simulink library "HANcoder_STM32_Target"  (R2018b)
settings: Solver=ode45  StartTime=0.0  StopTime=10.0  RelTol=1e-3  EnableMultiTasking=on
libraries: simulink x4
(part 3 of 9)

== system HANcoder_STM32_Target/Olimexino STM32 F3/PWM Outputs ==
  PWM Duty Cycle : Subsystem  Tag=HANcoder_TARGET_STM32_F3_Olimexino  mask(Pulse Width Modulation Set Duty Cycle){pinID=TIM1 - CON3 - D6, tsamp=-1}
      mask prompts: pinID "Output pin"; tsamp "Sample time"
      mask help:
      | Function
      | ========
      | A 'PWM Duty Cycle' block allows the duty cycle of the generated PWM signal to
      | changed.
      | Note that this only works properly if a 'PWM Init' block is also present
      | for initializing the related PWM module.
      |
      | Parameters
      | ==========
      | PWM pin:
      |   Selects the PWM pin for which the duty cycle should be updated.
      |
      | Inport
      | ==========
      | uint16 10-bit unsigned value (0..1023) to represent the duty cycle (0..100%) for
      | each enabled channel.
      mask init:
      | pinIDInfoStr = sfcn_pwmout_setduty_mcb(1, pinID);
      settings: MoveFcn=drawLogos
      mask Help: web('sfcn_pwmout_setduty.html');
      mask TypeOptions pinID: TIM1 - CON3 - D6 | TIM1 - CON3 - D7 | TIM1 - CON4 - D8 | TIM2 - CON3 - D2 | TIM2 - CON3 - D3 | TIM2 - CON3 - D0 | TIM3 - EXT - D35 | TIM3 - EXT - D36 | TIM3 - EXT - D37 | TIM4 - CON3 - D5 | TIM4 - CON4 - D9 | TIM4 - CON4 - D14 | TIM4 - EXT - D24
      mask Display: fprintf('PWM Set Duty Cycle\n%s', pinIDInfoStr);patch([129 148 147 128],[2 6 10 6],[0.89804 0 0.33725]);
  PWM Frequency : Subsystem  Tag=HANcoder_TARGET_STM32_F3_Olimexino  mask(Pulse Width Modulation Set Frequency){timID=TIM1, tsamp=-1}
      mask prompts: timID "Select a timer"; tsamp "Sample time"
      mask help:
      | Function
      | ========
      | A 'PWM Frequency' block allows the frequency of the generated PWM signal to change.
      | Note that this only works properly if a 'PWM Init' block is also present for initializing the related PWM module.
      |
      | Parameters
      | ==========
      | TIM:
      |   Selects the timer for which the frequency should be updated.
      |
      | Inport
      | ==========
      | A value that represents the new frequency [Hz]
      mask init:
      | timIDInfoStr = sfcn_pwmout_setfrequency_mcb(1, timID);
      settings: MoveFcn=drawLogos
      mask Help: web('sfcn_pwmout_setfrequency.html');
      mask TypeOptions timID: TIM1 | TIM2 | TIM3 | TIM4
      mask Display: fprintf('PWM Set frequency\n%s', timIDInfoStr);patch([129 148 147 128],[2 6 10 6],[0.89804 0 0.33725]);
  PWM Init : Subsystem  Tag=HANcoder_TARGET_STM32_F3_Olimexino  mask(Pulse Width Modulation Initialization){moduleID=TIM1: D6 & D7 & D8 & n/a + N-channels D32 & D33 & D34, frequency=5022, alignment=Edge aligned, enableIRQoutput=off, ch1On=off, ch1Pol=Active high, ch1Inv=off, ch2On=off, ch2Pol=Active high, ch2Inv=off, ch3On=off, ch3Pol=Active high, ch3Inv=off, ch4On=off, ch4Pol=Active high, ch4Inv=off}
      mask prompts: moduleID "PWM module"; frequency "Signal frequency [Hz]"; alignment "Signal alignment"; enableIRQoutput "Enable IRQ output"; ch1On "Generate PWM signal on channel 1"; ch1Pol "Select signal polarity"; ch1Inv "Enable inverted signal on additional output pin"; ch2On "Generate PWM signal on channel 2"; ch2Pol "Select signal polarity"; ch2Inv "Enable inverted signal on additional output pin"; ch3On "Generate PWM signal on channel 3"; ch3Pol "Select signal polarity"; ch3Inv "Enable inverted signal on additional output pin"; ch4On "Generate PWM signal on channel 4"; ch4Pol "Select signal polarity"; ch4Inv "Enable inverted signal on additional output pin"
      mask help:
      | Function
      | ========
      | A 'PWM Init' block configures one of the STM32 timer modules for PWM
      | functionality, allowing a PWM signal to be generated on up to 4 timer
      | channels and their associated output pins.
      |
      | Parameters
      | ==========
      | General - PWM module:
      |   Select the PWM module to use. The name in the combo box contains
      |   information about which pins on the target belong to this timer module.
      |   Also the first pin corresponds with the first channel and so on:
      |   TIMx: Ch1 & Ch2 & Ch3...
      |
      | General - Signal frequency:
      |   Determines the signal frequency in Hz. If you click 'Apply' after entering
      |   the desired frequency it will automatically be adjusted to the closest
      |   supported value.
      |
      | General - Signal Aligment:
      |   Determines the aligment of the signal. It can either be edge aligned or
      |   center aligned.
      |
      | General - Enable IRQ output
      |   Controls whether or not the IRQ output is available.
      |
      | Channel x - Generate PWM signal on channel x:
      |   Enable to configure the channel for PWM functionality so that the PWM signal
      |   is outputted on the channel's associated microcontroller pin.
      |
      | Channel x - Signal polarity:
      |   Selects the polarity of the signal.
      |
      | Channel x - Enable inverted signal on additional output pin:
      |   When enabled, a second PWM signal will be generated on an additional
      |   microcontroller pin where the signal is an exact inversion of the first signal.
      mask init:
      | moduleIDInfoStr = sfcn_pwmout_init_mcb(1, moduleID, frequency, alignment, enableIRQoutput, ch1On, ch2On, ch3On, ch4On, ch1Pol, ch2Pol, ch3Pol, ch4Pol, ch1Inv, ch2Inv, ch3Inv, ch4Inv);
      settings: CopyFcn=sfcn_pwmout_init_chk();  MoveFcn=drawLogos
      mask Help: web('sfcn_pwmout_init.html');
      mask TypeOptions moduleID: TIM1: D6 & D7 & D8 & n/a + N-channels D32 & D33 & D34  | TIM2: D2 & D3 & n/a & D0 | TIM3: D35 & D36 & D37 & n/a | TIM4: D5 & D9 & D14 & D24
      mask Callback moduleID: sfcn_pwmout_init_chk();
      mask TypeOptions alignment: Edge aligned | Center aligned
      mask TypeOptions ch1Pol: Active high | Active low
      mask TypeOptions ch2Pol: Active high | Active low
      mask TypeOptions ch3Pol: Active high | Active low
      mask TypeOptions ch4Pol: Active high | Active low
      mask Display: fprintf('PWM Init\n%s', moduleIDInfoStr);patch([214 233 232 213],[2 6 10 6],[0.89804 0 0.33725]);

== system HANcoder_STM32_Target/Olimexino STM32 F3/SPI ==
  SPI master init : Subsystem  Tag=HANcoder_TARGET_STM32_F3_Olimexino  mask(SPI master init){channel=SPI1: D13 & D12 & D11, speed=9000 kHz, polarity=Idle low, phase=Sample bit on 1st clock edge}
      mask prompts: speed "Communication speed"
      mask help:
      | Function
      | ==========
      | Initialized a SPI master channel.
      |
      | Parameters per channel
      | ======================
      | - Select channel (SCK MISO MOSI)
      | - Select communication speed
      | - Select clock signal polarity
      | - Select clock phase to sample a bit
      mask init:
      | spiChannelInfoStr = sfcn_spi_master_init_mcb(1, channel, speed, polarity, phase);
      settings: CopyFcn=sfcn_spi_master_init_chk();  MoveFcn=drawLogos
      mask Help: web('sfcn_spi_master_init.html')
      mask TypeOptions channel: SPI1: D13 & D12 & D11 | SPI2: D32 & D33 & D34
      mask Callback channel: sfcn_spi_master_init_chk();
      mask TypeOptions speed: 36000 kHz | 18000 kHz | 9000 kHz | 4500 kHz | 2250 kHz | 1125 kHz | 562.5 kHz | 281.25 kHz
      mask TypeOptions polarity: Idle low | Idle high
      mask TypeOptions phase: Sample bit on 1st clock edge | Sample bit on 2nd clock edge
      mask Display: fprintf('SPI master init\n%s', spiChannelInfoStr);patch([205 224 223 204],[2 6 10 6],[0.89804 0 0.33725]);
  SPI master transfer : Subsystem  Tag=HANcoder_TARGET_STM32_F3_Olimexino  Priority=1  mask(SPI master transfer){channel=SPI1: D13 & D12 & D11, useSS=off, SSpin=CON2 - A0, SSenable=on, SSdisable=on, delayCycles=0, userPriority=1, tsamp=-1}
      mask prompts: useSS "Use slave select output"; SSpin "Slave select output pin"; SSenable "Enable slave select before transfer"; SSdisable "Disable slave select after transfer"; delayCycles "Delay cycles between slave select enable and transfer"; userPriority "Priority (use to set order of byte transfer, lowest number is executed first)"; tsamp "Sample time"
      mask help:
      | Function
      | ==========
      | Performs a byte transfer via SPI.
      |
      | Parameters per channel
      | ======================
      | - Select channel
      | - Select if a Slave Select output should be controlled
      |   * Select the Slave Select digital output pin
      |   * Select if the Slave Select should be made logic low before the transfer
      |   * Select if the Slave Select should be made logic high after the transfer
      |   * Enter the number of CPU cycles to delay between Slave Select enable and the transfer
      |
      | Inputs
      | ======
      | The byte value to send to the slave.
      |
      | Outputs
      | =======
      | The byte value received from the slave.
      mask init:
      | spiChannelInfoStr = sfcn_spi_master_transfer_mcb(1, channel, useSS, SSpin, SSenable, SSdisable, delayCycles);
      settings: MoveFcn=drawLogos
      mask Help: web('sfcn_spi_master_transfer.html')
      mask TypeOptions channel: SPI1: D13 & D12 & D11 | SPI2: D32 & D33 & D34
      mask Callback useSS:
      | % Get the mask parameter
      | useSS = get_param(gcb,'useSS');
      | 
      | if strcmp(useSS,'on')
      |     set_param(gcb,'MaskVisibilities',{'on','on','on','on','on','on','on','on'});
      | else
      |     set_param(gcb,'MaskVisibilities',{'on','on','off','off','off','off','on','on'});
      | end
      mask TypeOptions SSpin: CON2 - A0 | CON2 - A1 | CON2 - A2 | CON2 - A3 | CON2 - A4 | CON2 - A5 | CON3 - D0 | CON3 - D1 | CON3 - D2 | CON3 - D3/LED2 | CON3 - D4 | CON3 - D5 | CON3 - D6 | CON3 - D7 | CON4 - D8 | CON4 - D9 | CON4 - D10 | CON4 - D11 | CON4 - D12 | CON4 - D13/LED1 | EXT - D25 | EXT - D26 | EXT - D31 | EXT - D32 | EXT - D35 | EXT - D36 | EXT - D37
      mask Callback userPriority:
      | userPriority = get_param(gcb, 'userPriority');
      | set_param(gcb,'Priority',userPriority);
      mask Display: fprintf('SPI master transfer\n%s', spiChannelInfoStr);patch([204 223 222 203],[2 6 10 6],[0.89804 0 0.33725]);

== system HANcoder_STM32_Target/Olimexino STM32 F3/Servo ==
  Servo : Subsystem  Tag=HANcoder_TARGET_STM32_F3_Olimexino  mask(Servo){pinID=TIM2 - CON3 - D2, lowerLimit=1000, upperLimit=2000, tsamp=-1}
      mask prompts: pinID "Select a servo pin"; lowerLimit "Set lower limit for pulse width [us]"; upperLimit "Set upper limit for pulse width [us]"; tsamp "Sample time"
      mask help:
      | Function
      | ========
      | A 'Servo' block generates a PWM signal with a frequency of 50 Hz.
      | The pulse width can be changed between a lower limit (typically 1000 microseconds) and an upper limit (typically 2000 microseconds).
      |
      | Parameters
      | ==========
      | PWM pin:
      |   Selects the pin for which the PWM signal should be generated.
      |
      | Inport
      | ==========
      | A value in microseconds that sets the high time of the PWM pulse.
      | If the value is lower than the lower limit, it is set to the lower limit.
      | If the value is higher than the upper limit, it is set to the upper limit.
      mask init:
      | pinIDInfoStr = sfcn_servo_mcb(1, pinID, lowerLimit, upperLimit);
      settings: MoveFcn=drawLogos
      mask TypeOptions pinID: TIM1 - CON3 - D6 | TIM1 - CON3 - D7 | TIM1 - CON4 - D8 | TIM2 - CON3 - D2 | TIM2 - CON3 - D3 | TIM2 - CON3 - D0 | TIM3 - EXT - D35 | TIM3 - EXT - D36 | TIM3 - EXT - D37 | TIM4 - CON3 - D5 | TIM4 - CON4 - D9 | TIM4 - CON4 - D14 | TIM4 - EXT - D24
      mask Callback pinID: sfcn_servo_chk();
      mask DialogControl Limits Prompt: Limits
      mask Display: fprintf('Servo\n%s', pinIDInfoStr);patch([129 148 147 128],[2 6 10 6],[0.89804 0 0.33725]);

== system HANcoder_STM32_Target/Olimexino STM32 F3/System Config ==
  Base Sample Time config : Subsystem  Tag=HANcoder_TARGET_STM32_F3_Olimexino  Description=HANcoder Target STM32-Olimexino blockset version 1.2  mask(Base Sample Time config){baseSampleTime=10, extraStack=25}
      mask prompts: baseSampleTime "Define the base sample time [ms]"; extraStack "Additional task stack (bytes):"
      mask help:
      | Function
      | ==========
      | Sets the Base Sample Time in the model, and automatically sets the sample
      | time in the solver step time menu when the model is simulated or build.
      |
      | Parameters
      | ==========
      | Base Sample Time [milliseconds]
      | Default:    10[ms]
      | Min:        0.1[ms]
      |
      | Note: This is the only block where sample time is set in miliseconds,
      | all other blocks work with sample time in seconds
      |
      | It is possible to reserve extra stack space for the OS task that executes
      | the model on the embedded target (AppCtrlTask).
      mask init:
      | sfcn_base_sample_time_mcb(baseSampleTime*1000, extraStack,1);
      | HANcoderStruct = get_param(gcb,'UserData');
      | BlocksetVersion = HANcoderStruct.BlocksetVersion;
      settings: MoveFcn=drawLogos
      mask Help: web('sfcn_base_sample_time.html')
      mask Display: fprintf('Blockset version %s\nBase Sample Time:\n %gms',BlocksetVersion,baseSampleTime);patch([85 104 103 84],[2 6 10 6],[0.89804 0 0.33725]);
  Build settings : Subsystem  Tag=HANcoder_TARGET_STM32_F3_Olimexino  mask(Build Settings){AutoASAP2add=on, AutoFlash=USB}
      mask prompts: AutoASAP2add "Add signals and parameters automatically"; AutoFlash "Automatic flash after build"
      mask help:
      | Function
      | ==========
      | Auto Add:
      | Here you can turn the automatic adding of Signals and Parameters on or off. If the option is on all the parameters and signals which are not defined in the workspace will be added. You will be prompted for the value.
      |
      | Auto Flash:
      | This option will automatically start MicroBoot with the selected interface.
      settings: MoveFcn=drawLogos
      mask Help: web('build_settings.html')
      mask TypeOptions AutoASAP2add: on | off
      mask TypeOptions AutoFlash: off | USB-F3
      mask DialogControl ParameterTabVar0 Prompt: Auto Add
      mask DialogControl Control3 Prompt: With this option the undefined parameters and signals will automatically be added to the workspace for use with HANtune. You will be prompted for the parameter values.
      mask DialogControl ParameterTabVar01 Prompt: Auto Flash
      mask DialogControl Control2 Prompt: With this option you can choose to automatically start MicroBoot after the build is complete. MicroBoot will start flashing using the selected interface.
      mask Display: fprintf('Build settings\nAuto Add: %s\nAuto Flash: %s',AutoASAP2add, AutoFlash);patch([108 127 126 107],[2 6 10 6],[0.89804 0 0.33725]);
  CAN config : Subsystem  Tag=HANcoder_TARGET_STM32_F3_Olimexino  mask(CAN config){canBus1=on, baudRate1=500, rxMask1=hex2dec('00000000'), rxCode1=hex2dec('00000000'), rxMode1=Receive only 11-bit message identifiers, txBufSize1=32, evBufSize1=8}
      mask prompts: canBus1 "Use CAN bus"; baudRate1 "Baudrate CAN bus [kbit/s]"; rxMask1 "Reception filter Mask CAN bus"; rxCode1 "Reception filter Code CAN bus"; rxMode1 "Reception filter Mode CAN bus"; txBufSize1 "Transmit buffer size CAN bus (max 256)"; evBufSize1 "Event buffer size CAN bus (max 16)"
      mask help:
      | Function
      | ==========
      | Configures the settings for the STM32's CAN busses.
      |
      | Parameters per channel
      | ======================
      | - Activate channel
      | - Select baud rate (default 500[kbit/s])
      | - Select reception acceptance filter Code
      | - Select reception acceptance filter Mask
      | - Select reception acceptance filter Mode
      mask init:
      | sfcn_can_config_mcb(txBufSize1, evBufSize1, canBus1, baudRate1, rxMask1, rxCode1, rxMode1, 0, 1, 0, 0, 1);
      settings: MoveFcn=drawLogos
      mask Help: web('sfcn_can_config.html')
      mask TypeOptions baudRate1: 125 | 250 | 500 | 1000
      mask TypeOptions rxMode1: Receive only 11-bit message identifiers | Receive only 29-bit message identifiers | Received both 11- and 29-bit message identifiers
      mask DialogControl ParameterTabVar0 Prompt: CAN 1
      mask Display: fprintf('CAN1 : %x',canBus1);patch([52 71 70 51],[2 6 10 6],[0.89804 0 0.33725]);
  Custom ID config : Subsystem  Tag=HANcoder_TARGET_STM32_F3_Olimexino  mask(Custom ID config){softID=softwareID, softNUM=1}
      mask prompts: softID "Software ID Name"; softNUM "Software Version Number"
      mask help:
      | Function:
      | =========
      | This block can be used to override the generated software ID as the
      | current software version which is used for identification purposes.
      | It can also be used to add a version number behind the software ID.
      |
      | Details:
      | ========
      | If only a software version number is filled in, a software ID will be
      | generated and the version number will be placed behind it.
      | At least one of the fields has to be filled in.
      |
      | Parameters:
      | ===========
      | Software ID name:
      | Fill in the desired custom ID.
      | Software Version Number:
      | Fill in the desired version number.
      mask init:
      | sfcn_custom_version_config_mcb(softID, softNUM)
      settings: MoveFcn=drawLogos
      mask Help: web('sfcn_custom_ID_config.html')
      mask Display: fprintf('Custom software ID:\n "%s"\n Software version:\n "%s"', char(softID), char(softNUM));patch([106 125 124 105],[2 6 10 6],[0.89804 0 0.33725]);
  XCP on CAN config : Subsystem  Tag=HANcoder_TARGET_STM32_F3_Olimexino  mask(XCP on CAN config){canBus=CAN 1, croID=hex2dec('665'), dtoID=hex2dec('666')}
      mask prompts: canBus "CAN channel"; croID "CRO identifier"; dtoID "DTO identifier"
      mask help:
      | Function
      | ==========
      | Implements XCP communication into your application.
      |
      | Parameter
      | ==========
      | Specify the CAN channel to be used for XCP.
      | Specify the CAN CRO message identifier for XCP (master->slave).
      | Specify the CAN DTO message identifier for XCP (slave->master).
      |
      | Notes
      | ==========
      | Baudrates can be modified in the CAN config block.
      mask init:
      | sfcn_can_xcp_config_mcb(canBus, croID, dtoID)
      settings: MoveFcn=drawLogos
      mask Help: web('sfcn_can_xcp_config.html')
      mask TypeOptions canBus: CAN 1
      mask Display: fprintf('XCP over CAN: %x',canBus);patch([63 82 81 62],[2 6 10 6],[0.89804 0 0.33725]);
  XCP on UART config : Subsystem  Tag=HANcoder_TARGET_STM32_F3_Olimexino  mask(XCP on UART config){channel=UART2: D1 & D0, baudrate=115200}
      mask prompts: channel "Select a channel"; baudrate "Select baudrate [bps]"
      mask help:
      | Function
      | ==========
      | Implements XCP communication into your application using the UART.
      mask init:
      | [uartChannelInfoStr, baudrateStr] = sfcn_uart_xcp_config_mcb(1, channel, baudrate);
      settings: MoveFcn=drawLogos
      mask TypeOptions channel: UART1: D7 & D8 | UART2: D1 & D0 | UART3: D29 & D30
      mask TypeOptions baudrate: 9600 | 19200 | 38400 | 57600 | 115200
      mask Display: fprintf('XCP over\n%s\n%s bps', uartChannelInfoStr, baudrateStr);patch([83 102 101 82],[2 6 10 6],[0.89804 0 0.33725]);
  XCP on USB config : Subsystem  Tag=HANcoder_TARGET_STM32_F3_Olimexino  mask(XCP on USB config){}
      mask help:
      | Function
      | ==========
      | Implements XCP communication into your application using the USB Virtual COM-port.
      mask init:
      | sfcn_usb_xcp_config_mcb()
      settings: MoveFcn=drawLogos
      mask Help: web('sfcn_usb_xcp_config.html')
      mask Display: fprintf('XCP over USB');patch([63 82 81 62],[2 6 10 6],[0.89804 0 0.33725]);

== system HANcoder_STM32_Target/Olimexino STM32 F3/System Management ==
  Enter Critical Section : Subsystem  Tag=HANcoder_TARGET_STM32_F3_Olimexino  mask(Enter a critical section){tsamp=-1}
      mask prompts: tsamp "Sample time"
      mask help:
      | Function
      | ==========
      | Enters a critical section that can not be interrupted. This block must
      | always be used in a pair together with "Exit Critical Section". Click the
      | Help-button for a detailed example on how to use this block.
      mask init:
      | sfcn_critical_enter_mcb();
      settings: MoveFcn=drawLogos
      mask Help: web('sfcn_critical_section.html');
      mask Display: fprintf('Enter Critical Section');patch([89 108 107 88],[2 6 10 6],[0.89804 0 0.33725]);
  Exit Critical Section : Subsystem  Tag=HANcoder_TARGET_STM32_F3_Olimexino  mask(Exit a critical section){tsamp=-1}
      mask prompts: tsamp "Sample time"
      mask help:
      | Function
      | ==========
      | Exits a critical section. This block must always be used in a pair together
      | with "Enter Critical Section". Click the Help-button for a detailed example
      | on how to use this block.
      mask init:
      | sfcn_critical_exit_mcb();
      settings: MoveFcn=drawLogos
      mask Help: web('sfcn_critical_section.html');
      mask Display: fprintf('Exit Critical Section');patch([89 108 107 88],[2 6 10 6],[0.89804 0 0.33725]);
  Get CPU load : Subsystem  Tag=HANcoder_TARGET_STM32_F3_Olimexino  mask(Get CPU load){mode=Current CPU load, tsamp=-1}
      mask prompts: tsamp "Sample time"
      mask help:
      | Function
      | ==========
      | Get the CPU load of the system.
      |
      | Parameters
      | ==========
      | Mode specifies if the current CPU load should be read or the maximum CPU
      | load since reset.
      |
      | Outport
      | ==========
      | CPU load as a percentage.
      mask init:
      | if mode==1
      |   modeStr = 'current';
      | else
      |   modeStr = 'maximum';
      | end
      | sfcn_controller_cpu_getload_mcb(mode);
      settings: MoveFcn=drawLogos
      mask Help: web('sfcn_controller_cpu_getload.html');
      mask TypeOptions mode: Current CPU load | Maximum CPU load
      mask Display: fprintf('Get %s\nCPU load', modeStr);patch([89 108 107 88],[2 6 10 6],[0.89804 0 0.33725]);
  Get free Heap : Subsystem  Tag=HANcoder_TARGET_STM32_F3_Olimexino  mask(Get free Heap){tsamp=-1}
      mask prompts: tsamp "Sample time"
      mask help:
      | Function
      | ==========
      | Obtains the number of bytes that are still available on the heap.
      |
      | Outport
      | ==========
      | Number of bytes that are still available on the heap.
      mask init:
      | sfcn_controller_getheap_mcb();
      settings: MoveFcn=drawLogos
      mask Help: web('sfcn_controller_getheap.html');
      mask Display: fprintf('Get free Heap');patch([89 108 107 88],[2 6 10 6],[0.89804 0 0.33725]);
  Get free Stack : Subsystem  Tag=HANcoder_TARGET_STM32_F3_Olimexino  mask(Get free Stack){taskIdx=Application Control Task, tsamp=-1}
      mask prompts: taskIdx "Task name"; tsamp "Sample time"
      mask help:
      | Function
      | ========
      | Obtains the number of bytes that are still available on the stack of a particular task.
      |
      | Parameter
      | =========
      | Name of the task for which the free stack space should be read.
      |
      | Outport
      | =======
      | Number of bytes that are still available on the task's stack.
      mask init:
      | sfcn_controller_getstack_mcb(taskIdx);
      settings: MoveFcn=drawLogos
      mask Help: web('sfcn_controller_getstack.html');
      mask TypeOptions taskIdx: Idle Task | Timer Task | Can Event Task | Can Transmit Task | Application Control Task
      mask Display: fprintf('Get free Stack');patch([89 108 107 88],[2 6 10 6],[0.89804 0 0.33725]);
  Reset ECU : Subsystem  Tag=HANcoder_TARGET_STM32_F3_Olimexino  mask(Reset ECU){}
      mask help:
      | Function
      | ==========
      | Triggering this block causes the ECU to reset.
      mask init:
      | sfcn_controller_reset_mcb()
      settings: MoveFcn=drawLogos
      mask Help: web('sfcn_controller_reset.html');
      mask Display: fprintf('Reset ECU');patch([54 73 72 53],[2 6 10 6],[0.89804 0 0.33725]);

== system HANcoder_STM32_Target/Olimexino STM32 F3/Timer Inputs ==
  Quadrature Encoder Get : Subsystem  Tag=HANcoder_TARGET_STM32_F3_Olimexino  mask(Quadrature Encoder Inputs){moduleID=TIM1: D6 & D7 - 5V Tolerant, config=Floating, counterReset=off, tsamp=-1}
      mask prompts: moduleID "Quad encoder module"; config "Configuration"; counterReset "Show counter reset input"; tsamp "Sample time"
      mask help:
      | Function
      | ========
      | Reads the counter of the quadrature encoder module.
      |
      | Parameters
      | ==========
      | Quadrature encoder module:
      |   Selects the quadrature encoder module. The channel A and B signals of the
      |   encoder should be connected to the 2 input pins that belong to the module.
      |
      | Configuration:
      |   Determines if the input is floating or is connected to an internal
      |   pull-up or pull-down resistor.
      |
      | Show counter reset input:
      |   Configures if the input port for the counter reset should be shown.
      |
      |
      | Outport
      | ==========
      | 32-bit signed counter. The counter starts at zero and counts up or down
      | depending on the direction of the motor.
      mask init:
      | moduleIDInfoStr = sfcn_quad_encoder_get_mcb(1,moduleID, counterReset, config);
      settings: CopyFcn=sfcn_quad_encoder_get_chk();  MoveFcn=drawLogos
      mask Help: web('sfcn_quad_encoder_get.html');
      mask TypeOptions moduleID: TIM1: D6 & D7 - 5V Tolerant | TIM2: D2 & D3 | TIM3: D35 & D36 - 5V Tolerant | TIM4: D5 & D9 - 5V Tolerant
      mask Callback moduleID: sfcn_quad_encoder_get_chk();
      mask TypeOptions config: Floating | Pullup | Pulldown
      mask Display: fprintf('Quad Encoder Get\n%s', moduleIDInfoStr);patch([129 148 147 128],[2 6 10 6],[0.89804 0 0.33725]);
  Timer Input Get : Subsystem  Tag=HANcoder_TARGET_STM32_F3_Olimexino  mask(Timer Input Get){pin=TIM1: CON3 - D6 - 5V Tolerant, zeroHzTimeoutMs=2000, tsamp=-1}
      mask prompts: pin "Timer input pin"; zeroHzTimeoutMs "0 Hz detection time (ms)"; tsamp "Sample time"
      mask help:
      | Function
      | ========
      | Reads the information from a timer input pin.
      |
      | Parameters
      | ==========
      | Timer input pin:
      |   Selects the timer input pin.
      |
      | Zero Hz detection time:
      |   Determines after how many milliseconds since the last edge the 0 Hz
      |   detected output flag should go high.
      |
      | Outport
      | ==========
      | Frequency
      |   The last measured frequency on the pin in Hz.
      |
      | Duty cycle
      |   The last measured duty cycle on the pin as a % with a scaling factor of 100 for
      |   improved resolution. So 5000 = 50% for example.
      |
      | Edge count
      |   The number of edges that were detected on the input pin since startup.
      |
      | Edge timestamp
      |   A 32-bit timestamp value of the last edge. The timestamp is derived from an
      |   internal 32-bit free running counter that runs at 24 Mhz.
      |
      | 0 Hz detected
      |   A boolean flag that will go high if no edges were detected for the time specified
      |   as the zero Hz detection time. Upon the next edge the flag will go low again.
      mask init:
      | timeinPinIdInfoStr = sfcn_timein_get_mcb(1, pin, zeroHzTimeoutMs);
      settings: CopyFcn=sfcn_timein_get_chk();  MoveFcn=drawLogos
      mask Help: web('sfcn_timein_get.html');
      mask TypeOptions pin: TIM1: CON3 - D6 - 5V Tolerant | TIM1: CON3 - D7 - 5V Tolerant | TIM1: CON4 - D8 - 5V Tolerant | TIM2: CON3 - D2 | TIM2: CON3 - D3 | TIM2: CON3 - D1 | TIM2: CON3 - D0 | TIM3: EXT - D35 - 5V Tolerant | TIM3: EXT - D36 - 5V Tolerant | TIM3: EXT - D37 - 5V Tolerant | TIM4: CON3 - D5 - 5V Tolerant | TIM4: CON4 - D9 - 5V Tolerant | TIM4: CON4 - D14 - 5V Tolerant | TIM4: EXT - D24 - 5V Tolerant
      mask Callback pin: sfcn_timein_get_chk();
      mask Display:
      | fprintf('Timer Input Get\n%s', timeinPinIdInfoStr);
      | port_label('output', 1, 'Frequency');
      | port_label('output', 2, 'Duty cycle');
      | port_label('output', 3, 'Edge count');
      | port_label('output', 4, 'Edge state');
      | port_label('output', 5, 'Edge timestamp');
      | port_label('output', 6, 'Counter timestamp');
      | port_label('output', 7, '0 Hz detected');patch([254 273 272 253],[2 6 10 6],[0.89804 0 0.33725]);
  Timer Input IRQ : Subsystem  Tag=HANcoder_TARGET_STM32_F3_Olimexino  mask(Timer Input IRQ){pin=TIM1: CON3 - D6 - 5V Tolerant}
      mask prompts: pin "Timer input pin"
      mask help:
      | Function
      | ========
      | Enables a function call subsystem to be connected that is executed on interrupt level
      | each time an edge change on the input pin was detected.
      |
      | Parameters
      | ==========
      | Timer input pin:
      |   Selects the timer input pin.
      |
      | Outport
      | =======
      | IRQ
      |   Allows connection of a function call subsystem.
      mask init:
      | timeinPinIdInfoStr = sfcn_timein_irq_mcb(1, pin);
      settings: CopyFcn=sfcn_timein_irq_chk();  MoveFcn=drawLogos
      mask Help: web('sfcn_timein_irq.html');
      mask TypeOptions pin: TIM1: CON3 - D6 - 5V Tolerant | TIM1: CON3 - D7 - 5V Tolerant | TIM1: CON4 - D8 - 5V Tolerant | TIM2: CON3 - D2 | TIM2: CON3 - D3 | TIM2: CON3 - D1 | TIM2: CON3 - D0 | TIM3: EXT - D35 - 5V Tolerant | TIM3: EXT - D36 - 5V Tolerant | TIM3: EXT - D37 - 5V Tolerant | TIM4: CON3 - D5 - 5V Tolerant | TIM4: CON4 - D9 - 5V Tolerant | TIM4: CON4 - D14 - 5V Tolerant | TIM4: EXT - D24 - 5V Tolerant
      mask Callback pin: sfcn_timein_irq_chk();
      mask Display: fprintf('Timer Input IRQ\n%s', timeinPinIdInfoStr);patch([244 263 262 243],[2 6 10 6],[0.89804 0 0.33725]);

== system HANcoder_STM32_Target/Olimexino STM32 F3/Timer Outputs ==
  Compare Event IRQ : Subsystem  Tag=HANcoder_TARGET_STM32_F3_Olimexino  mask(Compare Event IRQ){pin=TIM1: CON3 - D6 - 5V Tolerant}
      mask prompts: pin "Timer output pin"
      mask help:
      | Function
      | ========
      | Enables a function call subsystem to be connected that is executed on interrupt
      | level each time an output compare event was triggered.
      |
      | Parameters
      | ==========
      | Timer Output Pin:
      |   Selects the timer channel.
      |
      | Outport
      | =======
      | IRQ
      |   Allows connection of a function call subsystem.
      mask init:
      | timeoutPinIdInfoStr = sfcn_timeout_event_irq_mcb(1, pin);
      settings: CopyFcn=sfcn_timeout_event_irq_chk();  MoveFcn=drawLogos
      mask Help: web('sfcn_timeout_event_irq.html');
      mask TypeOptions pin: TIM1: CON3 - D6 - 5V Tolerant | TIM1: CON3 - D7 - 5V Tolerant | TIM1: CON4 - D8 - 5V Tolerant | TIM2: CON3 - D2 | TIM2: CON3 - D3 | TIM2: CON3 - D1 | TIM2: CON3 - D0 | TIM3: EXT - D35 - 5V Tolerant | TIM3: EXT - D36 - 5V Tolerant | TIM3: EXT - D37 - 5V Tolerant | TIM4: CON3 - D5 - 5V Tolerant | TIM4: CON4 - D9 - 5V Tolerant | TIM4: CON4 - D14 - 5V Tolerant | TIM4: EXT - D24 - 5V Tolerant
      mask Callback pin: sfcn_timeout_event_irq_chk();
      mask Display: fprintf('Compare Event IRQ\n%s', timeoutPinIdInfoStr);patch([129 148 147 128],[2 6 10 6],[0.89804 0 0.33725]);
  Get Free Running Counter : Subsystem  Tag=HANcoder_TARGET_STM32_F3_Olimexino  mask(Get Free Running Counter){moduleID=TIM1: D6 & D7 & D8 & n/a, tsamp=-1}
      mask prompts: moduleID "Timer module"; tsamp "Sample time"
      mask help:
      | Function
      | ========
      | Reads the timer module's internal 16-bit free running counter value.
      |
      | Parameters
      | ==========
      | Timer Module:
      |   Selects the timer module.
      |
      | Outport
      | =======
      | 16-bit free running counter value.
      mask init:
      | moduleIDInfoStr = sfcn_timeout_getrunningcounter_mcb(1, moduleID);
      settings: MoveFcn=drawLogos
      mask Help: web('sfcn_timeout_getrunningcounter.html');
      mask TypeOptions moduleID: TIM1: D6 & D7 & D8 & n/a | TIM2: D2 & D3 & D1 & D0 | TIM3: D35 & D36 & D37 & n/a | TIM4: D5 & D9 & D14 & D24
      mask Display: fprintf('Get Free Running Counter\n%s', moduleIDInfoStr);patch([129 148 147 128],[2 6 10 6],[0.89804 0 0.33725]);
  Get Last Event Counter : Subsystem  Tag=HANcoder_TARGET_STM32_F3_Olimexino  mask(Get Last Event Counter){pin=TIM1: CON3 - D6 - 5V Tolerant, tsamp=-1}
      mask prompts: pin "Timer output pin"; tsamp "Sample time"
      mask help:
      | Function
      | ========
      | Reads the timer channel's timestamp of the 16-bit free running counter
      | value at which the last output compare event occurred.
      |
      | Parameters
      | ==========
      | Timer Output Pin:
      |   Selects the timer channel.
      |
      | Outport
      | =======
      | 16-bit free running counter timestamp of the last output compare event.
      mask init:
      | timeoutPinIdInfoStr = sfcn_timeout_getlasteventcounter_mcb(1, pin);
      settings: MoveFcn=drawLogos
      mask Help: web('sfcn_timeout_getlasteventcounter.html');
      mask TypeOptions pin: TIM1: CON3 - D6 - 5V Tolerant | TIM1: CON3 - D7 - 5V Tolerant | TIM1: CON4 - D8 - 5V Tolerant | TIM2: CON3 - D2 | TIM2: CON3 - D3 | TIM2: CON3 - D1 | TIM2: CON3 - D0 | TIM3: EXT - D35 - 5V Tolerant | TIM3: EXT - D36 - 5V Tolerant | TIM3: EXT - D37 - 5V Tolerant | TIM4: CON3 - D5 - 5V Tolerant | TIM4: CON4 - D9 - 5V Tolerant | TIM4: CON4 - D14 - 5V Tolerant | TIM4: EXT - D24 - 5V Tolerant
      mask Display: fprintf('Get Last Event Counter\n%s', timeoutPinIdInfoStr);patch([129 148 147 128],[2 6 10 6],[0.89804 0 0.33725]);
  Output Compare Init : Subsystem  Tag=HANcoder_TARGET_STM32_F3_Olimexino  mask(Output Compare Init){moduleID=TIM1: D6 & D7 & D8 & n/a, frequency=2000000, enableIRQoutput=off}
      mask prompts: moduleID "Timer module"; frequency "Frequency (free running counter) [Hz]"; enableIRQoutput "Enable IRQ output"
      mask help:
      | Function
      | ========
      | Initializes the timer module to allow output compare functionality on the
      | module's channels.
      |
      | Parameters
      | ==========
      | Timer Module:
      |   Selects the timer module.
      |
      | Frequency:
      |   Frequency at which the 16-bit free running counter counts.
      |
      | Enable IRQ output
      |   Controls whether or not the IRQ output is available.
      |
      | Outport
      | =======
      | IRQ
      |   Allows connection of a function call subsystem for the free running
      |   counter overflow event.
      mask init:
      | moduleIDInfoStr = sfcn_timeout_init_mcb(1, moduleID, frequency, enableIRQoutput);
      settings: CopyFcn=sfcn_timeout_init_chk();  MoveFcn=drawLogos
      mask Help: web('sfcn_timeout_init.html');
      mask TypeOptions moduleID: TIM1: D6 & D7 & D8 & n/a | TIM2: D2 & D3 & D1 & D0 | TIM3: D35 & D36 & D37 & n/a | TIM4: D5 & D9 & D14 & D24
      mask Callback moduleID: sfcn_timeout_init_chk();
      mask Display: fprintf('Output Compare Init\n%s', moduleIDInfoStr);patch([129 148 147 128],[2 6 10 6],[0.89804 0 0.33725]);
  Reset Free Running Counter : Subsystem  Tag=HANcoder_TARGET_STM32_F3_Olimexino  mask(Reset Free Running Counter){moduleID=TIM1: D6 & D7 & D8 & n/a}
      mask prompts: moduleID "Timer module"
      mask help:
      | Function
      | ========
      | Resets the value of the timer module's 16-bit free running counter back to
      | 0.
      |
      | Triggerport
      | ===========
      | Connect the port to a trigger source to execute the block only when necessary.
      mask init:
      | moduleIDInfoStr = sfcn_timeout_resetcounter_mcb(1, moduleID);
      settings: MoveFcn=drawLogos
      mask Help: web('sfcn_timeout_resetcounter.html');
      mask TypeOptions moduleID: TIM1: D6 & D7 & D8 & n/a | TIM2: D2 & D3 & D1 & D0 | TIM3: D35 & D36 & D37 & n/a | TIM4: D5 & D9 & D14 & D24
      mask Display: fprintf('Reset Free Running Counter\n%s', moduleIDInfoStr);patch([126 145 144 125],[2 6 10 6],[0.89804 0 0.33725]);
  Schedule Compare Event : Subsystem  Tag=HANcoder_TARGET_STM32_F3_Olimexino  mask(Schedule Compare Event){pin=TIM1: CON3 - D6 - 5V Tolerant, tsamp=-1}
      mask prompts: pin "Timer output pin"; tsamp "Sample time"
      mask help:
      | Function
      | ========
      | Schedules the next output compare event. The first input determines the
      | value of the timer module's 16-bit free running counter when the event
      | should trigger. The second input determines the action that should
      | be taken on the timer channel's pin.
      |
      | Parameters
      | ==========
      | Timer output pin:
      |   Selects the timer channel's pin.
      |
      | Inport
      | ======
      | Counter
      |   Value of the timer module's 16-bit free running counter at which the
      |   event should trigger.
      |
      | Action
      |   Action to take on the channel's pin when the event triggers:
      |   0: set output pin to logic low.
      |   1: set output pin to logic high.
      |   2: invert logic state of the outpin pin.
      |   3: do nothing to the output pin.
      mask init:
      | timeoutPinIdInfoStr = sfcn_timeout_scheduleevent_mcb(1, pin);
      settings: MoveFcn=drawLogos
      mask Help: web('sfcn_timeout_scheduleevent.html');
      mask TypeOptions pin: TIM1: CON3 - D6 - 5V Tolerant | TIM1: CON3 - D7 - 5V Tolerant | TIM1: CON4 - D8 - 5V Tolerant | TIM2: CON3 - D2 | TIM2: CON3 - D3 | TIM2: CON3 - D1 | TIM2: CON3 - D0 | TIM3: EXT - D35 - 5V Tolerant | TIM3: EXT - D36 - 5V Tolerant | TIM3: EXT - D37 - 5V Tolerant | TIM4: CON3 - D5 - 5V Tolerant | TIM4: CON4 - D9 - 5V Tolerant | TIM4: CON4 - D14 - 5V Tolerant | TIM4: EXT - D24 - 5V Tolerant
      mask Display: fprintf('Schedule Compare Event\n%s', timeoutPinIdInfoStr);patch([129 148 147 128],[2 6 10 6],[0.89804 0 0.33725]);

== system HANcoder_STM32_Target/Olimexino STM32 F3/UART ==
  UART init : Subsystem  Tag=HANcoder_TARGET_STM32_F3_Olimexino  mask(UART init){channel=UART1: D7 & D8, baudrate=19200, databits=8, parity=none, stopbits=1, txbufsize=32, rxbufsize=32, useStatusOut=off}
      mask prompts: baudrate "Baudrate (bit/s)"; txbufsize "Transmit buffer size"; rxbufsize "Receive buffer size"; useStatusOut "Use status output"
      mask help:
      | Function
      | ==========
      | Initialized a UART channel.
      |
      | Parameters per channel
      | ======================
      | - Select channel
      | - Select baudrate
      | - Select number of databits
      | - Select parity
      | - Select number of stopbits
      | - Configure the size of the transmit buffer
      | - Configure the size of the reception buffer
      | - Enable/disable the status output port
      mask init:
      | uartChannelInfoStr = sfcn_uart_init_mcb(1, channel, baudrate, databits, parity, stopbits, txbufsize, rxbufsize, useStatusOut);
      settings: CopyFcn=sfcn_uart_init_chk();  MoveFcn=drawLogos
      mask Help: web('sfcn_uart_init.html')
      mask TypeOptions channel: UART1: D7 & D8 | UART2: D1 & D0 | UART3: D29 & D30
      mask Callback channel: sfcn_uart_init_chk();
      mask TypeOptions baudrate: 300 | 600 | 1200 | 2400 | 4800 | 9600 | 19200 | 38400 | 57600 | 115200
      mask TypeOptions databits: 8 | 9
      mask TypeOptions parity: none | even | odd
      mask TypeOptions stopbits: 1 | 2
      mask Display: fprintf('UART init\n%s', uartChannelInfoStr);patch([155 174 173 154],[2 6 10 6],[0.89804 0 0.33725]);
  UART receive : Subsystem  Tag=HANcoder_TARGET_STM32_F3_Olimexino  mask(UART receive){channel=UART1: D7 & D8, useStatusOut=off, tsamp=-1}
      mask prompts: useStatusOut "Use status outport"; tsamp "Sample time"
      mask help:
      | Function
      | ==========
      | Reads a byte from the UART reception buffer.
      |
      | Parameters per channel
      | ======================
      | - Select channel
      | - Select if the status output should be enabled.
      |
      | Outputs
      | =======
      | - The value of the receive byte.
      | - When the status output is 0, the reception buffer was empty.
      mask init:
      | uartChannelInfoStr = sfcn_uart_receive_mcb(1, channel, useStatusOut);
      settings: MoveFcn=drawLogos
      mask Help: web('sfcn_uart_receive.html')
      mask TypeOptions channel: UART1: D7 & D8 | UART2: D1 & D0 | UART3: D29 & D30
      mask Display: fprintf('UART receive\n%s', uartChannelInfoStr);patch([154 173 172 153],[2 6 10 6],[0.89804 0 0.33725]);
  UART receive buffer status : Subsystem  Tag=HANcoder_TARGET_STM32_F3_Olimexino  mask(UART receive buffer status){channel=UART1: D7 & D8, tsamp=-1}
      mask prompts: tsamp "Sample time"
      mask help:
      | Function
      | ==========
      | Obtains the number of received bytes that are currently stored in the
      | reception buffer.
      |
      | Parameters per channel
      | ======================
      | - Select channel
      |
      | Outputs
      | ======
      | - The number of bytes currently stored in the reception buffer.
      mask init:
      | uartChannelInfoStr = sfcn_uart_receive_size_mcb(1, channel);
      settings: MoveFcn=drawLogos
      mask Help: web('sfcn_uart_receive_size.html')
      mask TypeOptions channel: UART1: D7 & D8 | UART2: D1 & D0 | UART3: D29 & D30
      mask Display: fprintf('UART receive buffer status\n%s', uartChannelInfoStr);patch([154 173 172 153],[2 6 10 6],[0.89804 0 0.33725]);
  UART send : Subsystem  Tag=HANcoder_TARGET_STM32_F3_Olimexino  mask(UART send){channel=UART1: D7 & D8, useStatusOut=off, tsamp=-1}
      mask prompts: useStatusOut "Use status outport"; tsamp "Sample time"
      mask help:
      | Function
      | ==========
      | Transmits a byte on the UART communication interface.
      |
      | Parameters per channel
      | ======================
      | - Select channel
      | - Select if the status output should be enabled.
      |
      | Inputs
      | ======
      | - The byte to send
      |
      | Outputs
      | =======
      | - When the status output is 0, the byte could not be transmitted. Probably
      |   because the transmit buffer was configured too small.
      mask init:
      | uartChannelInfoStr = sfcn_uart_send_mcb(1, channel, useStatusOut);
      settings: MoveFcn=drawLogos
      mask Help: web('sfcn_uart_send.html')
      mask TypeOptions channel: UART1: D7 & D8 | UART2: D1 & D0 | UART3: D29 & D30
      mask Display: fprintf('UART send\n%s', uartChannelInfoStr);patch([154 173 172 153],[2 6 10 6],[0.89804 0 0.33725]);

== system HANcoder_STM32_Target/Olimexino STM32 F3/UDS ==
  UDS Get Key : Subsystem  Tag=HANcoder_TARGET_STM32_F3_Olimexino  mask(UDS Get Key){tsamp=-1}
      mask prompts: tsamp "Sample time"
      mask help:
      | Function
      | ==========
      | Reads the 32-bit key value that was received from the UDS tester.
      |
      | Outport
      | =======
      |  - Key value that was received from the UDS tester.
      mask init:
      | sfcn_uds_get_key_mcb();
      settings: MoveFcn=drawLogos
      mask Help: web('sfcn_uds_get_key.html');
      mask Display: fprintf('UDS Get Key');patch([59 78 77 58],[2 6 10 6],[0.89804 0 0.33725]);
  UDS Get Seed : Subsystem  Tag=HANcoder_TARGET_STM32_F3_Olimexino  mask(UDS Get Seed){tsamp=-1}
      mask prompts: tsamp "Sample time"
      mask help:
      | Function
      | ==========
      | Reads the 32-bit seed value to be used in the seed/key unlock sequence.
      |
      | Outport
      | =======
      |  - Seed value to be used in the seed/key unlock sequence.
      mask init:
      | sfcn_uds_get_seed_mcb();
      settings: MoveFcn=drawLogos
      mask Help: web('sfcn_uds_get_seed.html');
      mask Display: fprintf('UDS Get Seed');patch([59 78 77 58],[2 6 10 6],[0.89804 0 0.33725]);
  UDS Get Seed Event : Subsystem  Tag=HANcoder_TARGET_STM32_F3_Olimexino  mask(UDS Get Seed Event){}
      mask help:
      | Function
      | ========
      | A 'UDS Get Seed Event' block is needed when the parameter 'UDS seed/key
      | required' is set to TRUE (checked) in the 'UDS Init' block.
      |
      | This block has a function call output that gets triggered during a seed/key
      | sequence, when the UDS module needs a seed. The connected subsystem should
      | contain a 'UDS Set Seed' block to give the seed back to the UDS module.
      |
      | Outport
      | =======
      | Event
      |   Allows connection of a function call subsystem.
      mask init:
      | sfcn_uds_get_seed_event_mcb();
      settings: MoveFcn=drawLogos
      mask Help: web('sfcn_uds_get_seed_event.html');
      mask Display: fprintf('UDS Get Seed Event');patch([89 108 107 88],[2 6 10 6],[0.89804 0 0.33725]);
  UDS Init : Subsystem  Tag=HANcoder_TARGET_STM32_F3_Olimexino  mask(UDS Init){canChannel=CAN 1, canTxId=hex2dec('7E8'), canRxId=hex2dec('7E0'), tpBlockSize=4, tpSTmin=40, tpRxBuffSize=64, udsTxBuffSize=64, udsUseSeedKey=off}
      mask prompts: canChannel "CAN channel"; canTxId "CAN transmit ID"; canRxId "CAN receive ID"; tpBlockSize "TP blocksize"; tpSTmin "TP STmin"; tpRxBuffSize "TP reception buffer size"; udsTxBuffSize "UDS transmit buffer size"; udsUseSeedKey "UDS seed/key required"
      mask help:
      | Function
      | ==========
      | Initializes the Unified Diagnostic Services (UDS) communication module.
      |
      | Parameters
      | ==========
      | CAN channel: The CAN channel to communicate on
      | CAN transmit ID: CAN identifier for ECU to Tester
      | CAN receive ID: CAN identifier for Tester to ECU
      | TP blocksize: Number of CF's to receive before sending a FC
      | TP STmin: Min separation time (ms) expected between CF's
      | TP reception buffer size: Size of the buffer for TP receptions
      | UDS transmit buffer size: Size of the buffer for UDS/TP transmissions
      | UDS seed/key required: Requires a seed/key unlock sequence
      mask init:
      | sfcn_uds_init_mcb(canChannel, canTxId, canRxId, tpBlockSize, tpSTmin, tpRxBuffSize, udsTxBuffSize, udsUseSeedKey);
      settings: MoveFcn=drawLogos
      mask Help: web('sfcn_uds_init.html');
      mask TypeOptions canChannel: CAN 1
      mask TypeOptions tpBlockSize: 1 | 2 | 3 | 4 | 5 | 6 | 7 | 8 | 9 | 10 | 11 | 12 | 13 | 14 | 15 | 16 | 17 | 18 | 19 | 20 | 21 | 22 | 23 | 24 | 25 | 26 | 27 | 28 | 29 | 30 | 31 | 32 | 33 | 34 | 35 | 36 | 37 | 38 | 39 | 40 | 41 | 42 | 43 | 44 | 45 | 46 | 47 | 48 | 49 | 50 | 51 | 52 | 53 | 54 | 55 | 56 | 57 | 58 | 59 | 60 | 61 | 62 | 63 | 64 | 65 | 66 | 67 | 68 | 69 | 70 | 71 | 72 | 73 | 74 | 75 | 76 | 77 | 78 | 79 | 80 | 81 | 82 | 83 | 84 | 85 | 86 | 87 | 88 | 89 | 90 | 91 | 92 | 93 | 94 | 95 | 96 | 97 | 98 | 99 | 100 | 101 | 102 | 103 | 104 | 105 | 106 | 107 | 108 | 109 | 110 | 111 | 112 | 113 | 114 | 115 | 116 | 117 | 118 | 119 | 120 | 121 | 122 | 123 | 124 | 125 | 126 | 127 | 128 | 129 | 130 | 131 | 132 | 133 | 134 | 135 | 136 | 137 | 138 | 139 | 140 | 141 | 142 | 143 | 144 | 145 | 146 | 147 | 148 | 149 | 150 | 151 | 152 | 153 | 154 | 155 | 156 | 157 | 158 | 159 | 160 | 161 | 162 | 163 | 164 | 165 | 166 | 167 | 168 | 169 | 170 | 171 | 172 | 173 | 174 | 175 | 176 | 177 | 178 | 179 | 180 | 181 | 182 | 183 | 184 | 185 | 186 | 187 | 188 | 189 | 190 | 191 | 192 | 193 | 194 | 195 | 196 | 197 | 198 | 199 | 200 | 201 | 202 | 203 | 204 | 205 | 206 | 207 | 208 | 209 | 210 | 211 | 212 | 213 | 214 | 215 | 216 | 217 | 218 | 219 | 220 | 221 | 222 | 223 | 224 | 225 | 226 | 227 | 228 | 229 | 230 | 231 | 232 | 233 | 234 | 235 | 236 | 237 | 238 | 239 | 240 | 241 | 242 | 243 | 244 | 245 | 246 | 247 | 248 | 249 | 250 | 251 | 252 | 253 | 254 | 255
      mask TypeOptions tpSTmin: 1 | 2 | 3 | 4 | 5 | 6 | 7 | 8 | 9 | 10 | 11 | 12 | 13 | 14 | 15 | 16 | 17 | 18 | 19 | 20 | 21 | 22 | 23 | 24 | 25 | 26 | 27 | 28 | 29 | 30 | 31 | 32 | 33 | 34 | 35 | 36 | 37 | 38 | 39 | 40 | 41 | 42 | 43 | 44 | 45 | 46 | 47 | 48 | 49 | 50 | 51 | 52 | 53 | 54 | 55 | 56 | 57 | 58 | 59 | 60 | 61 | 62 | 63 | 64 | 65 | 66 | 67 | 68 | 69 | 70 | 71 | 72 | 73 | 74 | 75 | 76 | 77 | 78 | 79 | 80 | 81 | 82 | 83 | 84 | 85 | 86 | 87 | 88 | 89 | 90 | 91 | 92 | 93 | 94 | 95 | 96 | 97 | 98 | 99 | 100 | 101 | 102 | 103 | 104 | 105 | 106 | 107 | 108 | 109 | 110 | 111 | 112 | 113 | 114 | 115 | 116 | 117 | 118 | 119 | 120 | 121 | 122 | 123 | 124 | 125 | 126 | 127 | 128 | 129 | 130 | 131 | 132 | 133 | 134 | 135 | 136 | 137 | 138 | 139 | 140 | 141 | 142 | 143 | 144 | 145 | 146 | 147 | 148 | 149 | 150 | 151 | 152 | 153 | 154 | 155 | 156 | 157 | 158 | 159 | 160 | 161 | 162 | 163 | 164 | 165 | 166 | 167 | 168 | 169 | 170 | 171 | 172 | 173 | 174 | 175 | 176 | 177 | 178 | 179 | 180 | 181 | 182 | 183 | 184 | 185 | 186 | 187 | 188 | 189 | 190 | 191 | 192 | 193 | 194 | 195 | 196 | 197 | 198 | 199 | 200 | 201 | 202 | 203 | 204 | 205 | 206 | 207 | 208 | 209 | 210 | 211 | 212 | 213 | 214 | 215 | 216 | 217 | 218 | 219 | 220 | 221 | 222 | 223 | 224 | 225 | 226 | 227 | 228 | 229 | 230 | 231 | 232 | 233 | 234 | 235 | 236 | 237 | 238 | 239 | 240 | 241 | 242 | 243 | 244 | 245 | 246 | 247 | 248 | 249 | 250 | 251 | 252 | 253 | 254 | 255
      mask Display: fprintf('UDS Init\n(CAN %x)', canChannel);patch([59 78 77 58],[2 6 10 6],[0.89804 0 0.33725]);
  UDS Set Key Verfied : Subsystem  Tag=HANcoder_TARGET_STM32_F3_Olimexino  mask(UDS Set Key Verified){tsamp=-1}
      mask prompts: tsamp "Sample time"
      mask help:
      | Function
      | ========
      | Informs the UDS module whether or not the key received from the UDS tester
      | is valid.
      |
      | Inport
      | ======
      |  - Set to TRUE in case the key was valid, FALSE otherwise.
      mask init:
      | sfcn_uds_set_key_verified_mcb();
      settings: MoveFcn=drawLogos
      mask Help: web('sfcn_uds_set_key_verified.html');
      mask Display: fprintf('UDS Set Key\nVerified');patch([59 78 77 58],[2 6 10 6],[0.89804 0 0.33725]);
  UDS Set Seed : Subsystem  Tag=HANcoder_TARGET_STM32_F3_Olimexino  mask(UDS Set Seed){tsamp=-1}
      mask prompts: tsamp "Sample time"
      mask help:
      | Function
      | ==========
      | Sets the 32-bit seed value to be used in the seed/key unlock sequence.
      |
      | Inport
      | ======
      |  - Seed value to be used in the seed/key unlock sequence.
      mask init:
      | sfcn_uds_set_seed_mcb();
      settings: MoveFcn=drawLogos
      mask Help: web('sfcn_uds_set_seed.html');
      mask Display: fprintf('UDS Set Seed');patch([59 78 77 58],[2 6 10 6],[0.89804 0 0.33725]);
  UDS Verify Key Event : Subsystem  Tag=HANcoder_TARGET_STM32_F3_Olimexino  mask(UDS Verify Key Event){}
      mask help:
      | Function
      | ========
      | A 'UDS Verify Key Event' block is needed when the parameter 'UDS seed/key
      | required' is set to TRUE (checked) in the 'UDS Init' block.
      |
      | This block has a function call output that gets triggered during a seed/key
      | sequence, when the UDS module received a 32-bit key from the tester that
      | needs to be verified. The connected subsystem should contain a 'UDS Set Key
      | Verfied' block to inform the UDS module if the received key was correct.
      |
      | Outport
      | =======
      | Event
      |   Allows connection of a function call subsystem.
      mask init:
      | sfcn_uds_verify_key_event_mcb();
      settings: MoveFcn=drawLogos
      mask Help: web('sfcn_uds_verify_key_event.html');
      mask Display: fprintf('UDS Verify Key Event');patch([89 108 107 88],[2 6 10 6],[0.89804 0 0.33725]);

== system HANcoder_STM32_Target/STM32-E407/Analog Inputs ==
  Analog Input : Subsystem  Tag=HANcoder_TARGET_STM32_E407  mask(Analog Input){pinID=CON2 - A1, tsamp=-1, filtered=off}
      mask prompts: pinID "Input pin"; tsamp "Sample time"; filtered "Use oversamping and filtering (causes high CPU load)"
      mask help:
      | Function
      | ========
      | Reads the analog/digital conversion results of an analog input pin.
      |
      | Parameters
      | ==========
      | Input pin:
      |   Selects the analog input to read
      |
      | Outport
      | ==========
      | uint16 12-bit conversion results (0-4095).
      mask init:
      | pinIDInfoStr = sfcn_analog_in_mcb(2, pinID,filtered);
      settings: MoveFcn=drawLogos
      mask Help: web('sfcn_analog_in.html');
      mask TypeOptions pinID: CON PF - 6 | CON PF - 7 | CON PF - 8 | CON2 - A1 | CON2 - A2 | CON2 - A3 | CON2 - A4 | CON2 - A5 | CON2 - A0 | UEXT - 7
      mask Callback pinID:
      | BlockMaskValues = get_param(gcb, 'MaskValues');
      | HANcoderPinChecks(BlockMaskValues{1}, 'E407');
      | clear BlockMaskValues;
      mask Display: fprintf('Analog Input\n%s', pinIDInfoStr);patch([129 148 147 128],[2 6 10 6],[0.89804 0 0.33725]);

== system HANcoder_STM32_Target/STM32-E407/Analog Outputs ==
  Analog Output : Subsystem  Tag=HANcoder_TARGET_STM32_E407  mask(Analog Output){pinID=CON4 - D10, tsamp=-1}
      mask prompts: pinID "Output pin"; tsamp "Sample time"
      mask help:
      | Function
      | ========
      | Controls the state of an analog output pin.
      |
      | Parameters
      | ==========
      | Output pin:
      |   Selects the analog output to control
      |
      | Inport
      | ==========
      | [uint16] Output voltage 0-4095 (0-100%)
      mask init:
      | pinID = sfcn_analog_out_mcb(2,pinID);
      settings: CopyFcn=sfcn_digital_out_chk();  MoveFcn=drawLogos
      mask Help: web('sfcn_analog_out.html');
      mask TypeOptions pinID: CON4 - D10 | CON4 - D13
      mask Display: fprintf('Analog Output\n%s',pinID);patch([129 148 147 128],[2 6 10 6],[0.89804 0 0.33725]);

== system HANcoder_STM32_Target/STM32-E407/CAN ==
  CAN : Subsystem
      settings: MoveFcn=drawLogos
      mask Display: fprintf('CAN');patch([79 98 97 78],[2 6 10 6],[0.89804 0 0.33725]);
  CANopenNode : Subsystem
      settings: MoveFcn=drawLogos
      mask Display: fprintf('CANopenNode');patch([79 98 97 78],[2 6 10 6],[0.89804 0 0.33725]);
